simulink model "rlQubeServo_ours_angle"  (R2025a)
settings: Solver=ode23t  StartTime=0.0  StopTime=10.0  RelTol=1e-3  AbsTol=1e-3
values from neighbouring files (symbols this model uses):
  dphi0 = 0    [TrainAgentsToControlQuanserQUBEPendulumExample.m]    (also in sac.m; sac_ours_0.mat; sac_ours_angle_1.mat; sac_ours_angle_2_.mat)
  dtheta0 = 0    [TrainAgentsToControlQuanserQUBEPendulumExample.m]    (also in sac.m; sac_ours_0.mat; sac_ours_angle_1.mat; sac_ours_angle_2_.mat)
  phi0 = pi-pi/4+rand*pi/2    [TrainAgentsToControlQuanserQUBEPendulumExample.m]    (also in ppo.m = pi - pi/4 + rand * pi/2; sac.m = pi+(2*rand-1)*pi/4; sac_ours_0.mat = 0; sac_ours_angle_1.mat = 0)
  theta0 = -pi/4+rand*pi/2    [TrainAgentsToControlQuanserQUBEPendulumExample.m]    (also in ppo.m = -pi/4 + rand * pi/2; sac.m = (2*rand-1)*pi/2; sac_ours_0.mat = 0; sac_ours_angle_1.mat = 0)
  theta_limit = 5*pi/8    (= 1.96349540849)    [TrainAgentsToControlQuanserQUBEPendulumExample.m]    (also in ppo.m; sac.m; sac_ours_0.mat; sac_ours_angle_1.mat)
  Ts = 0.005    [TrainAgentsToControlQuanserQUBEPendulumExample.m]    (also in ppo.m = 0.01; sac.m = 0.02; sac_ours_0.mat = 0.01; sac_ours_angle_1.mat = 0.01)
  volt_limit = 12    [TrainAgentsToControlQuanserQUBEPendulumExample.m]    (also in ppo.m; sac.m = 10; sac_ours_0.mat; sac_ours_angle_1.mat)
libraries: QuanserQube x1, rllib x1, simulink x1
settings Model: SimulationMode=accelerator  Creator=The MathWorks, Inc.  LastModifiedBy=cusgadmin
settings SolverCC: AutoScaleAbsTol=off  MaxZcPerStep=1.0
settings DataIOCC: SaveOutput=off  SaveTime=off
settings DebuggingCC: UnconnectedInputMsg=warning  UnconnectedOutputMsg=warning  UnconnectedLineMsg=warning
settings ModelReferenceCC: EnableRefExpFcnMdlSchedulingChecks=on
settings RTWCC: GPUComputeCapability=3.5  DLArmComputeVersion=19.05
settings ExplorerConfigSet: SimMechanicsOpenEditorOnUpdate=off  InternalSimMechanicsExplorerSettings="<ExplorerConfiguration><canonicalview>default</canonicalview><AnimationSetting><BasePlaybackSpeed>1.0</BasePlaybackSpeed><PlaybackSpeedFactor>1.0</PlaybackSpeedFactor></AnimationSetting><TilePanel><TileInfo><Tiles Columns=\"1\" Count=\"1\" Rows=\"1\"><Column Weight=\"1\"/><Row Weight=\"1\"/><Tile Height=\"1\" Width=\"1\" X=\"0\" Y=\"0\"/></Tiles></TileInfo><SceneInfo><SceneViewer><BGColor><R>0.60000002384185791</R><G>0.60000002384185791</G><B>0.60000002384185791</B></BGColor><Camera><DoPerspective>on</DoPerspective><Position><X>0.334156231583514596</X><Y>0.107146061295956732</Y><Z>0.154419804164132285</Z></Position><Center><X>0.145480827141795971</X><Y>0.0537418892551446009</Y><Z>0.077934111254939889</Z></Center><Up><X>-0.332530024195597795</X><Y>-0.157027945704575345</Y><Z>0.929927958110882913</Z></Up><ViewLimDist>1</ViewLimDist><YLim>0.466307658154998583</YLim><XLim>0.535390274177961367</XLim></Camera></SceneViewer></SceneInfo></TilePanel><MechEditorPanel><Cameras><Camera><Id>Camera1</Id><Value><Name>Camera1</Name><NativeCamera><PositionKeyframeSet/><CenterKeyframeSet/><UpVectorKeyframeSet/></NativeCamera></Value></Camera></Cameras><GfxPanelCameraMap><MapElement CameraMLId=\"Camera1\" GfxPanelIndex=\"0\"/></GfxPanelCameraMap><VideoCreator><PlaybackSpeedRatio>1.0</PlaybackSpeedRatio><FrameRate>30</FrameRate><VideoFormat>Motion JPEG AVI</VideoFormat><FrameSize>auto</FrameSize></VideoCreator></MechEditorPanel></ExplorerConfiguration>"

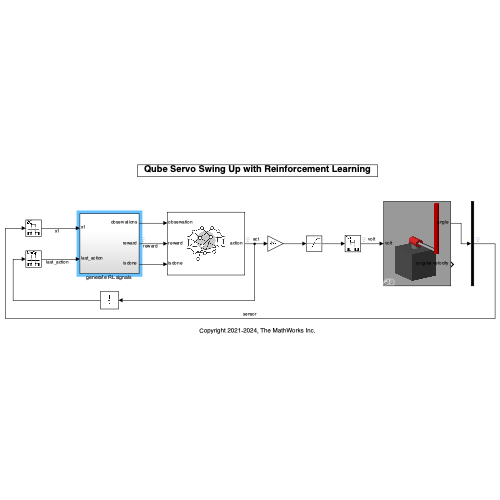
[thumbnail: Simulink's stored preview of the top-level diagram]
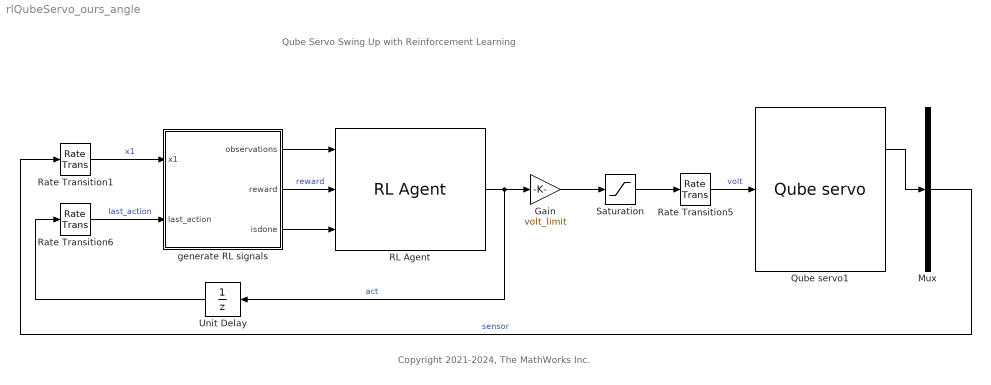
== system rlQubeServo_ours_angle ==
  note: Qube Servo Swing Up with Reinforcement Learning
  note: Copyright 2021-2024, The MathWorks Inc.
  Gain : Gain  Gain=volt_limit
  Mux : Mux  Inputs=1
  Qube servo1 : QuanserQube/Qube servo  a0=[theta0, phi0]  w0=[dtheta0,dphi0]  R_m=0.21  L_m=1.16e-3  mu_m=0.0024  K_b=0.07683  n=1  rod_mass=0.257  rod_length=0.216  rod_rad=0.01  p_mass=0.127  p_length=0.337  p_rad=0.005  D_r=0.28  D_p=0.00022  Choice_Stopper=On
  RL Agent : rllib/RL Agent  Agent=agent  ExternalActionAsInput=off  ProvideLastAction=off  ProvideCumRwd=off  TreatAsDirectFeedthrough=on  UseStrictObservationDataTypes=off
  Rate Transition1 : RateTransition  OutPortSampleTime=Ts
  Rate Transition5 : RateTransition
  Rate Transition6 : RateTransition  OutPortSampleTime=Ts
  Saturation : Saturate  UpperLimit=volt_limit  LowerLimit=-volt_limit
  Unit Delay : UnitDelay  SampleTime=-1  HasFrameUpgradeWarning=on
  generate RL signals : Subsystem
  wires:
  generate RL signals/3(isdone) -> RL Agent/3
  generate RL signals/2(reward) -> RL Agent/2  "reward"
  Qube servo1/1 -> Mux/1
  RL Agent/1 -> Gain/1, Unit Delay/1  "act"
  generate RL signals/1(observations) -> RL Agent/1
  Rate Transition1/1 -> generate RL signals/1(x1)  "x1"
  Unit Delay/1 -> Rate Transition6/1
  Mux/1 -> Rate Transition1/1  "sensor"
  Rate Transition6/1 -> generate RL signals/2(last_action)  "last_action"
  Saturation/1 -> Rate Transition5/1
  Rate Transition5/1 -> Qube servo1/1  "volt"
  Gain/1 -> Saturation/1

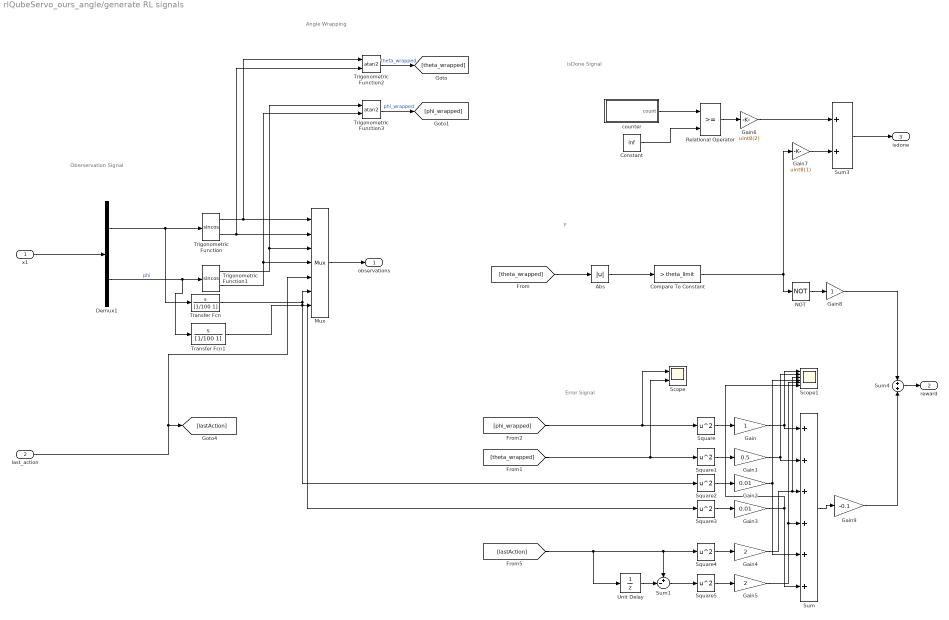
== system rlQubeServo_ours_angle/generate RL signals ==
  note: Oberservation Signal
  note: Error Signal
  note: isDone Signal
  note: Angle Wrapping
  note: F
  x1 : Inport  SampleTime=Ts
  last_action : Inport  Port=2
  Abs : Abs  SaturateOnIntegerOverflow=off
  Compare To Constant : simulink/Logic and Bit Operations/Compare To Constant  relop=>  const=theta_limit  OutDataTypeStr=boolean
  Constant : Constant  Value=inf
  Demux1 : Demux  Outputs=2
  Gain : Gain
  Gain1 : Gain  Gain=0.5
  Gain2 : Gain  Gain=0.01
  Gain3 : Gain  Gain=0.01
  Gain4 : Gain  Gain=2
  Gain5 : Gain  Gain=2
  Gain6 : Gain  Gain=uint8(2)  OutDataTypeStr=uint8
  Gain7 : Gain  Gain=uint8(1)  OutDataTypeStr=uint8
  Gain8 : Gain  OutDataTypeStr=double
  Gain9 : Gain  Gain=-0.1
  Mux : Mux  Inputs=7
  NOT : Logic  Operator=NOT  IconShape=distinctive  AllPortsSameDT=off  OutDataTypeStr=boolean
  Relational Operator : RelationalOperator  OutDataTypeStr=boolean  RndMeth=Simplest  InputSameDT=off
  Scope : Scope  NumInputPorts=2
      settings: ActiveDisplayYMinimum=-1  ActiveDisplayYMaximum=1
  Scope1 : Scope  NumInputPorts=6
      settings: ActiveDisplayYMinimum=-17.851137579386368  ActiveDisplayYMaximum=160.66023821447735
  Square{,1..5} (6 alike) : Math  Operator=square
  Sum : Sum  Inputs=++++++
  Sum1 : Sum  Inputs=+-|
  Sum3 : Sum
  Sum4 : Sum
  Transfer Fcn : TransferFcn  Numerator=[1 0]  Denominator=[1/100 1]
  Transfer Fcn1 : TransferFcn  Numerator=[1 0]  Denominator=[1/100 1]
  Trigonometric Function : Trigonometry  Operator=sincos
  Trigonometric Function1 : Trigonometry  Operator=sincos
  Trigonometric Function2 : Trigonometry  Operator=atan2
  Trigonometric Function3 : Trigonometry  Operator=atan2
  Unit Delay : UnitDelay  SampleTime=-1  HasFrameUpgradeWarning=on
  counter : Subsystem
  observations : Outport
  reward : Outport  Port=2
  isdone : Outport  Port=3
  wires:
  Trigonometric Function1/1 -> Trigonometric Function3/1, Mux/3
  Square1/1 -> Gain1/1
  Gain9/1 -> Sum4/2
  Unit Delay/1 -> Sum1/2
  Trigonometric Function2/1 -> [theta_wrapped]  "theta_wrapped"
  Mux/1 -> observations/1
  Trigonometric Function1/2 -> Mux/4, Trigonometric Function3/2
  Square5/1 -> Gain5/1
  Gain8/1 -> Sum4/1
  Square/1 -> Gain/1
  NOT/1 -> Gain8/1
  Square4/1 -> Gain4/1
  Gain1/1 -> Scope1/2, Sum/2
  Sum4/1 -> reward/1
  counter/1(count) -> Relational Operator/1
  Trigonometric Function/2 -> Trigonometric Function2/2, Mux/2
  x1/1 -> Demux1/1
  Relational Operator/1 -> Gain6/1
  Constant/1 -> Relational Operator/2
  Sum3/1 -> isdone/1
  Trigonometric Function/1 -> Trigonometric Function2/1, Mux/1
  Sum/1 -> Gain9/1
  Sum1/1 -> Square5/1
  Abs/1 -> Compare To Constant/1
  Gain/1 -> Scope1/1, Sum/1
  Demux1/1 -> Trigonometric Function/1, Transfer Fcn/1
  Demux1/2 -> Transfer Fcn1/1, Trigonometric Function1/1  "phi"
  [theta_wrapped] -> Abs/1
  last_action/1 -> Mux/5, [lastAction]
  [theta_wrapped] -> Scope/2, Square1/1
  Trigonometric Function3/1 -> [phi_wrapped]  "phi_wrapped"
  [phi_wrapped] -> Scope/1, Square/1
  [lastAction] -> Sum1/1, Square4/1, Unit Delay/1
  Gain6/1 -> Sum3/1
  Gain7/1 -> Sum3/2
  Gain4/1 -> Scope1/3, Sum/3
  Gain5/1 -> Scope1/5, Sum/4
  Transfer Fcn/1 -> Square2/1, Mux/6
  Transfer Fcn1/1 -> Square3/1, Mux/7
  Square2/1 -> Gain2/1
  Square3/1 -> Gain3/1
  Gain2/1 -> Scope1/4, Sum/5
  Gain3/1 -> Scope1/6, Sum/6
  Compare To Constant/1 -> NOT/1, Gain7/1

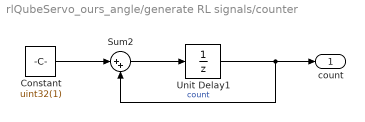
== system rlQubeServo_ours_angle/generate RL signals/counter ==
  Constant : Constant  Value=uint32(1)
  Sum2 : Sum  Inputs=|++
  Unit Delay1 : UnitDelay  SampleTime=Ts  HasFrameUpgradeWarning=on
  count : Outport  OutDataTypeStr=uint32
  wires:
  Sum2/1 -> Unit Delay1/1
  Unit Delay1/1 -> count/1, Sum2/2  "count"
  Constant/1 -> Sum2/1
